simulink model "AltitudeHold_PID_control"  (R2017a)
settings: Solver=VariableStepAuto  StartTime=0.0  StopTime=150  RelTol=1e-3
libraries: simulink x1
settings Model: Creator=Md Aadil  LastModifiedBy=Md Aadil

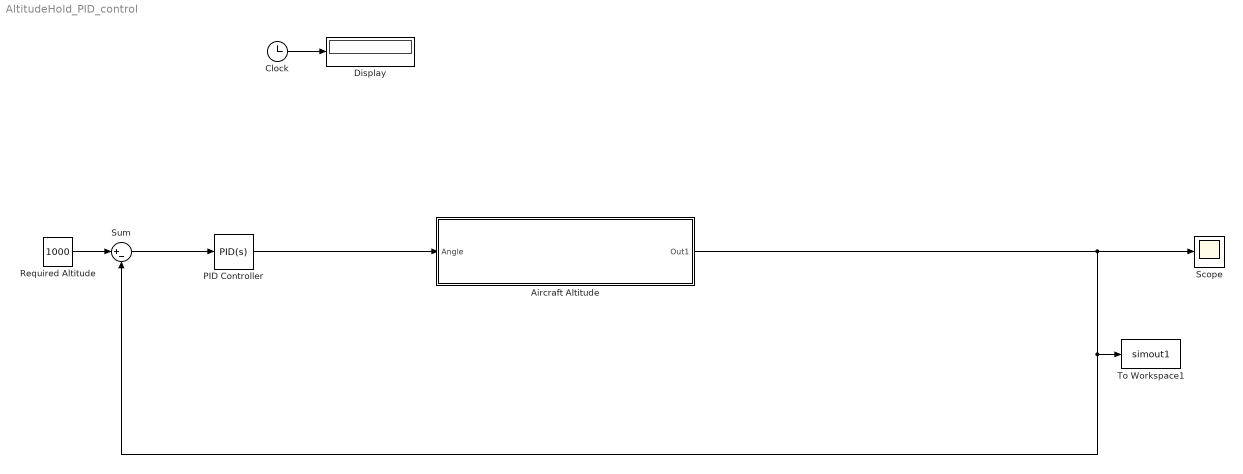
== system AltitudeHold_PID_control ==
  Aircraft Altitude : Subsystem  TreatAsAtomicUnit=on
  Clock : Clock
  Display : Display
  PID Controller : simulink/Continuous/PID Controller  Controller=PID  TimeDomain=Continuous-time  SampleTime=-1  IntegratorMethod=Forward Euler  FilterMethod=Forward Euler  Form=Parallel  UseFilter=on  ControllerParametersSource=internal  P=-0.03804263515044  I=-0.00176797955327235  D=-0.0942529009775036  N=217.761381573672  InitialConditionSource=internal  InitialConditionForIntegrator=0  InitialConditionForFilter=0  ExternalReset=none  LimitOutput=off  UpperSaturationLimit=inf  LowerSaturationLimit=-inf  LinearizeAsGain=on  AntiWindupMode=none  Kb=1  TrackingMode=off  Kt=1  PParamMin=[]  PParamMax=[]  IParamMin=[]  IParamMax=[]  DParamMin=[]  DParamMax=[]  NParamMin=[]  NParamMax=[]  KbParamMin=[]  KbParamMax=[]  KtParamMin=[]  KtParamMax=[]  POutMin=[]  POutMax=[]  IOutMin=[]  IOutMax=[]  DOutMin=[]  DOutMax=[]  NOutMin=[]  NOutMax=[]  KbOutMin=[]  KbOutMax=[]  KtOutMin=[]  KtOutMax=[]  IntegratorOutMin=[]  IntegratorOutMax=[]  FilterOutMin=[]  FilterOutMax=[]  SumOutMin=[]  SumOutMax=[]  SumI1OutMin=[]  SumI1OutMax=[]  SumI2OutMin=[]  SumI2OutMax=[]  SumI3OutMin=[]  SumI3OutMax=[]  SumDOutMin=[]  SumDOutMax=[]  SaturationOutMin=[]  SaturationOutMax=[]  IntegratorContinuousStateAttributes=''  IntegratorStateMustResolveToSignalObject=off  IntegratorRTWStateStorageClass=Auto  FilterContinuousStateAttributes=''  FilterStateMustResolveToSignalObject=off  FilterRTWStateStorageClass=Auto  DifferentiatorICPrevScaledInput=0  DifferentiatorOutMin=[]  DifferentiatorOutMax=[]  InitialConditionSetting=State (most efficient)
  "Required Altitude " : Constant  Value=1000
  Scope : Scope
  Sum : Sum  Inputs=|+-
  To Workspace1 : ToWorkspace  VariableName=simout1  SaveFormat=Timeseries  SampleTime=-1
  wires:
  "Required Altitude "/1 -> Sum/1
  Sum/1 -> PID Controller/1
  Clock/1 -> Display/1
  Aircraft Altitude/1(Out1) -> Sum/2, To Workspace1/1, Scope/1
  PID Controller/1 -> Aircraft Altitude/1(Angle)

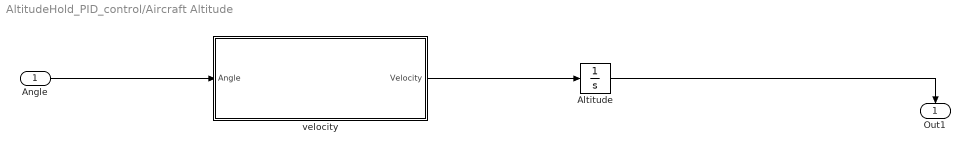
== system AltitudeHold_PID_control/Aircraft Altitude ==
  Angle : Inport
  " velocity" : Subsystem
  Altitude : Integrator  InitialCondition=500
  Out1 : Outport
  wires:
  Altitude/1 -> Out1/1
  Angle/1 -> " velocity"/1(Angle)
  " velocity"/1(Velocity) -> Altitude/1

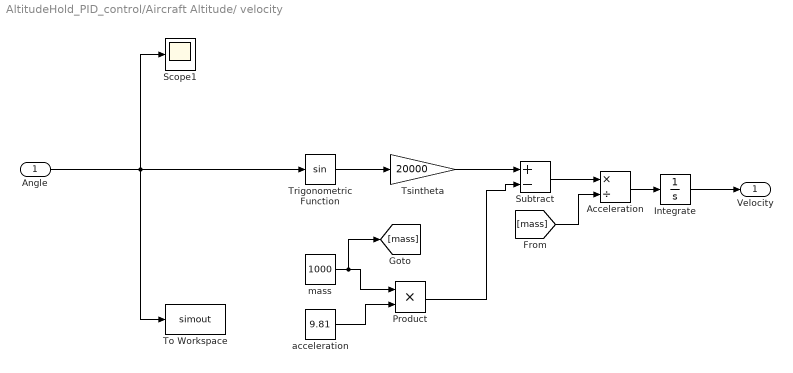
== system AltitudeHold_PID_control/Aircraft Altitude/ velocity ==
  Angle : Inport
  Acceleration : Product  Inputs=*/
  "Integrate " : Integrator
  Product : Product
  Scope1 : Scope
  Subtract : Sum  Inputs=+-
  To Workspace : ToWorkspace  VariableName=simout  SaveFormat=Timeseries  SampleTime=-1
  Trigonometric Function : Trigonometry
  "Tsintheta " : Gain  Gain=20000
  "acceleration " : Constant  Value=9.81
  mass : Constant  Value=1000
  Velocity : Outport
  wires:
  Acceleration/1 -> "Integrate "/1
  "acceleration "/1 -> Product/2
  "Tsintheta "/1 -> Subtract/1
  Angle/1 -> Trigonometric Function/1, To Workspace/1, Scope1/1
  Product/1 -> Subtract/2
  mass/1 -> [mass], Product/1
  Subtract/1 -> Acceleration/1
  "Integrate "/1 -> Velocity/1
  [mass] -> Acceleration/2
  Trigonometric Function/1 -> "Tsintheta "/1
